simulink model "cek_modelLevel"  (R2021b)
settings: Solver=VariableStepAuto  StartTime=0.0  StopTime=900  RelTol=1e-3
settings Model: Creator=Asus  LastModifiedBy=Asus

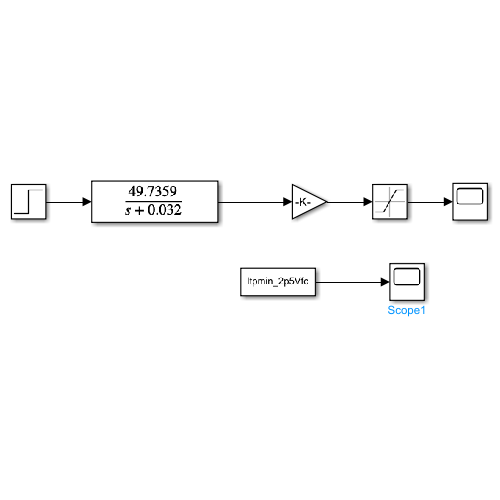
[thumbnail: Simulink's stored preview of the top-level diagram]
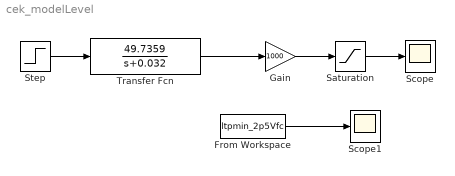
== system cek_modelLevel ==
  From Workspace : FromWorkspace  VariableName=ltpmin_2p5Vfc
  Gain : Gain  Gain=1000
  Saturation : Saturate  UpperLimit=240  LowerLimit=42
  Scope : Scope
  Scope1 : Scope
  Step : Step  After=0.000037169  SampleTime=0
  Transfer Fcn : TransferFcn  Numerator=[49.7359]  Denominator=[1 0.032]
  wires:
  Step/1 -> Transfer Fcn/1
  Transfer Fcn/1 -> Gain/1
  Gain/1 -> Saturation/1
  Saturation/1 -> Scope/1
  From Workspace/1 -> Scope1/1
